simulink model "Cv_04_2"  (R2022b)
settings: Solver=VariableStepAuto  StartTime=0.0  StopTime=10.0  RelTol=1e-3
values from neighbouring files (symbols this model uses):
  a0 = 2    [Cv_04_2m.m]
  a1 = 6    [Cv_04_2m.m]
  a2 = 8    [Cv_04_2m.m]
  a3 = 3    [Cv_04_2m.m]
  a4 = 1    [Cv_04_2m.m]
  b0 = 2    [Cv_04_2m.m]
settings Model: Creator=honza  LastModifiedBy=honza
settings DataIOCC: ReturnWorkspaceOutputs=off

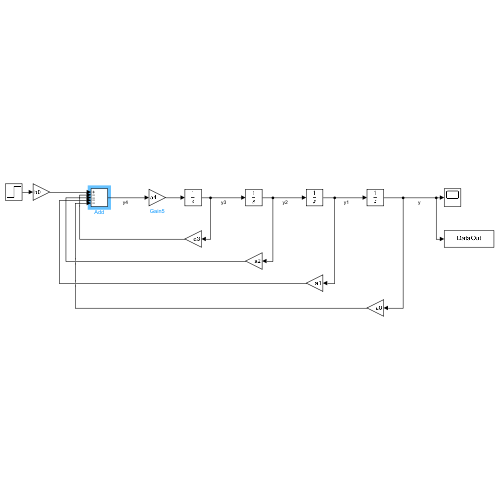
[thumbnail: Simulink's stored preview of the top-level diagram]
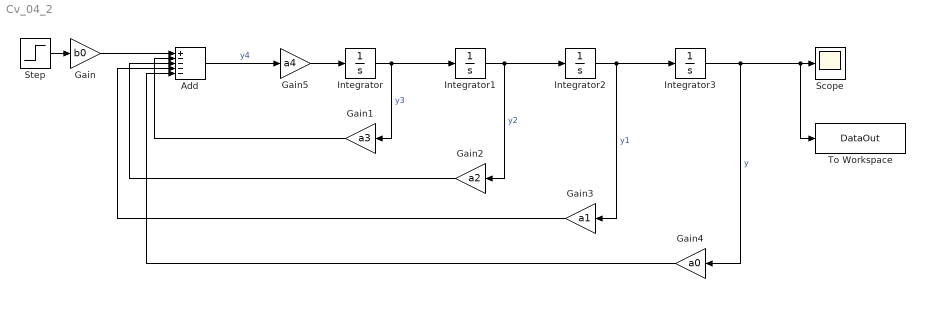
== system Cv_04_2 ==
  Add : Sum  Inputs=+----
  Gain : Gain  Gain=b0
  Gain1 : Gain  Gain=a3
  Gain2 : Gain  Gain=a2
  Gain3 : Gain  Gain=a1
  Gain4 : Gain  Gain=a0
  Gain5 : Gain  Gain=a4
  Integrator{,1..3} (4 alike) : Integrator
  Scope : Scope
  Step : Step  SampleTime=0
  To Workspace : ToWorkspace  VariableName=DataOut  SaveFormat=Timeseries  SampleTime=0.1
  wires:
  Integrator/1 -> Gain1/1, Integrator1/1  "y3"
  Integrator1/1 -> Gain2/1, Integrator2/1  "y2"
  Integrator2/1 -> Gain3/1, Integrator3/1  "y1"
  Integrator3/1 -> Gain4/1, To Workspace/1, Scope/1  "y"
  Add/1 -> Gain5/1  "y4"
  Step/1 -> Gain/1
  Gain/1 -> Add/1
  Gain1/1 -> Add/2
  Gain2/1 -> Add/3
  Gain3/1 -> Add/4
  Gain4/1 -> Add/5
  Gain5/1 -> Integrator/1
